simulink model "act_ut"  (Simulink 8.1)
settings: Solver=FixedStepDiscrete  StartTime=0.0  StopTime=100  FixedStep=0.005  RelTol=1e-3
libraries: siltestlib x3, act x1
settings Model: Creator=xsellart  LastModifiedBy=AT015555
settings DataIOCC: SignalLoggingSaveFormat=Dataset
settings OptimizationCC: ExpressionDepthLimit=128
settings DebuggingCC: FcnCallInpInsideContextMsg=EnableAllAsError
settings GRTTargetCC: CombineOutputUpdateFcns=on  GRTInterface=off

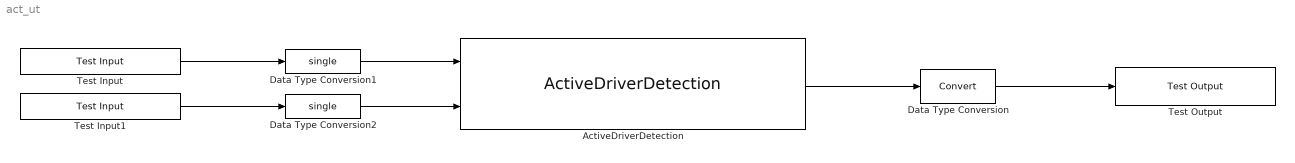
== system act_ut ==
  ActiveDriverDetection : act/ActiveDriverDetection
  Data Type Conversion : DataTypeConversion
  Data Type Conversion1 : DataTypeConversion  OutDataTypeStr=single
  Data Type Conversion2 : DataTypeConversion  OutDataTypeStr=single
  Test Input : siltestlib/Test Input  varname=VDINR_SteerSpeed_degps  sampletime=0.005
  Test Input1 : siltestlib/Test Input  varname=VDINR_HWAccelPedalPosn_pct  sampletime=0.005
  Test Output : siltestlib/Test Output  varname=VIFO_ActiveDriverDetec_flg  sampletime=-1
  wires:
  Test Input/1 -> Data Type Conversion1/1
  Data Type Conversion1/1 -> ActiveDriverDetection/1
  Test Input1/1 -> Data Type Conversion2/1
  Data Type Conversion2/1 -> ActiveDriverDetection/2
  ActiveDriverDetection/1 -> Data Type Conversion/1
  Data Type Conversion/1 -> Test Output/1
